simulink model "suspensions"  (R2021b)
settings: Solver=VariableStepAuto  StartTime=0.0  StopTime=10.0  RelTol=1e-3
values from neighbouring files (symbols this model uses):
  C = 1100    [suspension.m]
  k = 24000    [suspension.m]
  m = 700    [suspension.m]
settings Model: Creator=Madhav R  LastModifiedBy=Madhav R

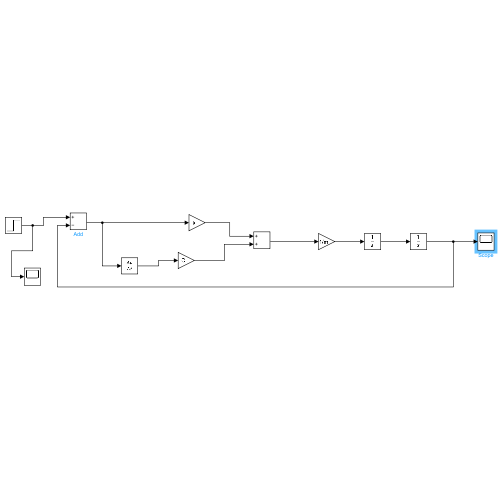
[thumbnail: Simulink's stored preview of the top-level diagram]
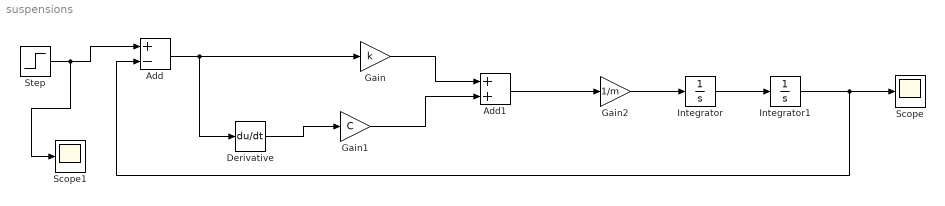
== system suspensions ==
  Add : Sum  Inputs=+-
  Add1 : Sum
  Derivative : Derivative
  Gain : Gain  Gain=k
  Gain1 : Gain  Gain=C
  Gain2 : Gain  Gain=1/m
  Integrator : Integrator
  Integrator1 : Integrator
  Scope : Scope
  Scope1 : Scope
  Step : Step  SampleTime=0
  wires:
  Step/1 -> Scope1/1, Add/1
  Add/1 -> Derivative/1, Gain/1
  Derivative/1 -> Gain1/1
  Gain1/1 -> Add1/2
  Gain/1 -> Add1/1
  Add1/1 -> Gain2/1
  Gain2/1 -> Integrator/1
  Integrator/1 -> Integrator1/1
  Integrator1/1 -> Add/2, Scope/1
